simulink model "Triangular_Comparator"  (R2020a)
settings: Solver=VariableStepAuto  StartTime=0.0  StopTime=0.01  RelTol=1e-3
settings Model: Creator=Harsh sachan  LastModifiedBy=Harsh sachan

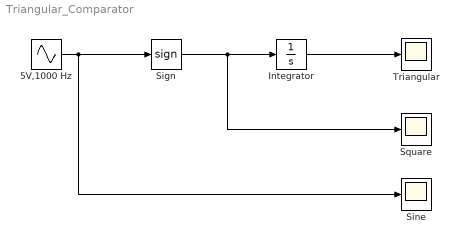
== system Triangular_Comparator ==
  5V,1000 Hz : Sin  Amplitude=5  Frequency=2*pi*1000  SampleTime=0
  Integrator : Integrator
  Sign : Signum
  "Sine " : Scope
  Square : Scope
  Triangular : Scope
  wires:
  Sign/1 -> Square/1, Integrator/1
  Integrator/1 -> Triangular/1
  5V,1000 Hz/1 -> "Sine "/1, Sign/1
